simulink library "ammclib_bam_s32k14x"  (Simulink 9.0)
settings: Solver=ode45  StartTime=0.0  StopTime=10.0  RelTol=1e-3
undefined symbols (not defined in the file): f16A1, f16A2, f16B0, f16B1, f16B2, f16C1, f16CC1, f16CC1sc, f16CC1sc_D, f16CC1sc_Q, f16CC1scD, f16CC1scQ, f16CC2, f16CC2sc, f16CC2sc_D, f16CC2sc_Q, f16CC2scD, f16CC2scQ, f16DerivGain, f16EGain, f16FiltCoef, f16HystOff, f16HystOn, f16IGain, f16IntegGain, f16IntegGainFW, f16IntegGainQ, f16Kd, f16Kq, f16Limit, f16LowerLim, f16LowerLimit_D, f16LowerLimit_Q, f16ModIndex, f16OutValOff, f16OutValOn, f16PropGain, f16PropGainFW, f16PropGainQ, f16RampDown, f16RampUp, f16UGain, f16UpperLim, f16UpperLimit, f16UpperLimit_D, f16UpperLimit_Q, f16WIGain, f32A1, f32A2, f32B0, f32B1, f32B2, f32C1, f32CC1, f32CC1sc, f32CC1sc_D, f32CC1sc_Q, f32CC1scD, f32CC1scQ, f32CC2 ... (+122)
(part 10 of 11)

== system ammclib_bam_s32k14x/MLIB/bam_flt/MLIB_Mul_FLT ==
  note: ---------------------------------------------------------------------------------------------------------------------------------------------------------------------------------------------------
  fltIn1 : Inport
  fltIn2 : Inport  Port=2
  MLIB_Mul_SF : S-Function  FunctionName=MLIB_Mul_SF_FLT  SFunctionDeploymentMode=off  EnableBusSupport=off
  copyright : Subsystem
      mask Display:
      | text(10,90,'FILE:');text(10,75,'DESRIPTION:')
      | text(10,60,'COPYRIGHT:')
      | text(10,45,'VERSION:')
      | text(10,30,'DATE:')
  copyright2 : Subsystem
      mask Display:
      | text(10,90,'MLIB_Mul_BAM_FLT.mdl');text(10,75,'Sum of two input values.');text(10,60,'NXP')
      | text(10,45,'0.1');text(10,30,'26-Jul-2011');
  logo : Subsystem
      mask Display: image(imread('logo.jpg'))
  fltOut : Outport
  wires:
  MLIB_Mul_SF/1 -> fltOut/1
  fltIn2/1 -> MLIB_Mul_SF/2
  fltIn1/1 -> MLIB_Mul_SF/1

== system ammclib_bam_s32k14x/MLIB/bam_flt/MLIB_Neg_FLT ==
  note: ---------------------------------------------------------------------------------------------------------------------------------------------------------------------------------------------------
  fltIn : Inport
  MLIB_Neg_SF : S-Function  FunctionName=MLIB_Neg_SF_FLT  SFunctionDeploymentMode=off  EnableBusSupport=off
  copyright : Subsystem
      mask Display:
      | text(10,90,'FILE:');text(10,75,'DESRIPTION:')
      | text(10,60,'COPYRIGHT:')
      | text(10,45,'VERSION:')
      | text(10,30,'DATE:')
  copyright2 : Subsystem
      mask Display:
      | text(10,90,'MLIB_Neg_BAM_FLT.mdl');text(10,75,'Sum of two input values.');text(10,60,'NXP')
      | text(10,45,'0.1');text(10,30,'20-Jan-2012');
  logo : Subsystem
      mask Display: image(imread('logo.jpg'))
  fltOut : Outport
  wires:
  MLIB_Neg_SF/1 -> fltOut/1
  fltIn/1 -> MLIB_Neg_SF/1

== system ammclib_bam_s32k14x/MLIB/bam_flt/MLIB_Sub_FLT ==
  note: ---------------------------------------------------------------------------------------------------------------------------------------------------------------------------------------------------
  fltIn1 : Inport
  fltIn2 : Inport  Port=2
  MLIB_Sub_SF : S-Function  FunctionName=MLIB_Sub_SF_FLT  SFunctionDeploymentMode=off  EnableBusSupport=off
  copyright : Subsystem
      mask Display:
      | text(10,90,'FILE:');text(10,75,'DESRIPTION:')
      | text(10,60,'COPYRIGHT:')
      | text(10,45,'VERSION:')
      | text(10,30,'DATE:')
  copyright2 : Subsystem
      mask Display:
      | text(10,90,'MLIB_Sub_BAM_FLT.mdl');text(10,75,'Sum of two input values.');text(10,60,'NXP')
      | text(10,45,'0.1');text(10,30,'18-Jul-2011');
  logo : Subsystem
      mask Display: image(imread('logo.jpg'))
  fltOut : Outport
  wires:
  MLIB_Sub_SF/1 -> fltOut/1
  fltIn2/1 -> MLIB_Sub_SF/2
  fltIn1/1 -> MLIB_Sub_SF/1

== system ammclib_bam_s32k14x/MLIB/bam_flt/MLIB_VMac_FLT ==
  note: ---------------------------------------------------------------------------------------------------------------------------------------------------------------------------------------------------
  fltIn1 : Inport
  fltIn2 : Inport  Port=2
  fltIn3 : Inport  Port=3
  fltIn4 : Inport  Port=4
  MLIB_VMac_SF : S-Function  FunctionName=MLIB_VMac_SF_FLT  SFunctionDeploymentMode=off  EnableBusSupport=off
  copyright : Subsystem
      mask Display:
      | text(10,90,'FILE:');text(10,75,'DESRIPTION:')
      | text(10,60,'COPYRIGHT:')
      | text(10,45,'VERSION:')
      | text(10,30,'DATE:')
  copyright2 : Subsystem
      mask Display:
      | text(10,90,'MLIB_VMac_BAM_FLT.mdl');text(10,75,'Vector multiply accumulate.');text(10,60,'Freescale')
      | text(10,45,'0.1');text(10,30,'25-Aug-2011');
  logo : Subsystem
      mask Display: image(imread('logo.jpg'))
  fltOut : Outport
  wires:
  MLIB_VMac_SF/1 -> fltOut/1
  fltIn4/1 -> MLIB_VMac_SF/4
  fltIn3/1 -> MLIB_VMac_SF/3
  fltIn2/1 -> MLIB_VMac_SF/2
  fltIn1/1 -> MLIB_VMac_SF/1

== system ammclib_bam_s32k14x/AMCLIB/bam_f16/AMCLIB_BemfObsrvDQ_F16/copyright ==

== system ammclib_bam_s32k14x/AMCLIB/bam_f16/AMCLIB_BemfObsrvDQ_F16/copyright2 ==

== system ammclib_bam_s32k14x/AMCLIB/bam_f16/AMCLIB_BemfObsrvDQ_F16/logo ==

== system ammclib_bam_s32k14x/AMCLIB/bam_f16/AMCLIB_CurrentLoop_F16/copyright ==

== system ammclib_bam_s32k14x/AMCLIB/bam_f16/AMCLIB_CurrentLoop_F16/copyright2 ==

== system ammclib_bam_s32k14x/AMCLIB/bam_f16/AMCLIB_CurrentLoop_F16/logo ==

== system ammclib_bam_s32k14x/AMCLIB/bam_f16/AMCLIB_FWSpeedLoop_F16/copyright ==

== system ammclib_bam_s32k14x/AMCLIB/bam_f16/AMCLIB_FWSpeedLoop_F16/copyright2 ==

== system ammclib_bam_s32k14x/AMCLIB/bam_f16/AMCLIB_FWSpeedLoop_F16/logo ==

== system ammclib_bam_s32k14x/AMCLIB/bam_f16/AMCLIB_FW_F16/copyright ==

== system ammclib_bam_s32k14x/AMCLIB/bam_f16/AMCLIB_FW_F16/copyright2 ==

== system ammclib_bam_s32k14x/AMCLIB/bam_f16/AMCLIB_FW_F16/logo ==

== system ammclib_bam_s32k14x/AMCLIB/bam_f16/AMCLIB_SpeedLoop_F16/copyright ==

== system ammclib_bam_s32k14x/AMCLIB/bam_f16/AMCLIB_SpeedLoop_F16/copyright2 ==

== system ammclib_bam_s32k14x/AMCLIB/bam_f16/AMCLIB_SpeedLoop_F16/logo ==

== system ammclib_bam_s32k14x/AMCLIB/bam_f16/AMCLIB_TrackObsrv_F16/copyright ==

== system ammclib_bam_s32k14x/AMCLIB/bam_f16/AMCLIB_TrackObsrv_F16/copyright2 ==

== system ammclib_bam_s32k14x/AMCLIB/bam_f16/AMCLIB_TrackObsrv_F16/logo ==

== system ammclib_bam_s32k14x/AMCLIB/bam_f32/AMCLIB_BemfObsrvDQ_F32/copyright ==

== system ammclib_bam_s32k14x/AMCLIB/bam_f32/AMCLIB_BemfObsrvDQ_F32/copyright2 ==

== system ammclib_bam_s32k14x/AMCLIB/bam_f32/AMCLIB_BemfObsrvDQ_F32/logo ==

== system ammclib_bam_s32k14x/AMCLIB/bam_f32/AMCLIB_CurrentLoop_F32/copyright ==

== system ammclib_bam_s32k14x/AMCLIB/bam_f32/AMCLIB_CurrentLoop_F32/copyright2 ==

== system ammclib_bam_s32k14x/AMCLIB/bam_f32/AMCLIB_CurrentLoop_F32/logo ==

== system ammclib_bam_s32k14x/AMCLIB/bam_f32/AMCLIB_FWSpeedLoop_F32/copyright ==

== system ammclib_bam_s32k14x/AMCLIB/bam_f32/AMCLIB_FWSpeedLoop_F32/copyright2 ==

== system ammclib_bam_s32k14x/AMCLIB/bam_f32/AMCLIB_FWSpeedLoop_F32/logo ==

== system ammclib_bam_s32k14x/AMCLIB/bam_f32/AMCLIB_FW_F32/copyright ==

== system ammclib_bam_s32k14x/AMCLIB/bam_f32/AMCLIB_FW_F32/copyright2 ==

== system ammclib_bam_s32k14x/AMCLIB/bam_f32/AMCLIB_FW_F32/logo ==

== system ammclib_bam_s32k14x/AMCLIB/bam_f32/AMCLIB_SpeedLoop_F32/copyright ==

== system ammclib_bam_s32k14x/AMCLIB/bam_f32/AMCLIB_SpeedLoop_F32/copyright2 ==

== system ammclib_bam_s32k14x/AMCLIB/bam_f32/AMCLIB_SpeedLoop_F32/logo ==

== system ammclib_bam_s32k14x/AMCLIB/bam_f32/AMCLIB_TrackObsrv_F32/copyright ==

== system ammclib_bam_s32k14x/AMCLIB/bam_f32/AMCLIB_TrackObsrv_F32/copyright2 ==

== system ammclib_bam_s32k14x/AMCLIB/bam_f32/AMCLIB_TrackObsrv_F32/logo ==

== system ammclib_bam_s32k14x/AMCLIB/bam_flt/AMCLIB_BemfObsrvDQ_FLT/copyright ==

== system ammclib_bam_s32k14x/AMCLIB/bam_flt/AMCLIB_BemfObsrvDQ_FLT/copyright2 ==

== system ammclib_bam_s32k14x/AMCLIB/bam_flt/AMCLIB_BemfObsrvDQ_FLT/logo ==

== system ammclib_bam_s32k14x/AMCLIB/bam_flt/AMCLIB_CurrentLoop_FLT/copyright ==

== system ammclib_bam_s32k14x/AMCLIB/bam_flt/AMCLIB_CurrentLoop_FLT/copyright2 ==

== system ammclib_bam_s32k14x/AMCLIB/bam_flt/AMCLIB_CurrentLoop_FLT/logo ==

== system ammclib_bam_s32k14x/AMCLIB/bam_flt/AMCLIB_FWSpeedLoop_FLT/copyright ==

== system ammclib_bam_s32k14x/AMCLIB/bam_flt/AMCLIB_FWSpeedLoop_FLT/copyright2 ==

== system ammclib_bam_s32k14x/AMCLIB/bam_flt/AMCLIB_FWSpeedLoop_FLT/logo ==

== system ammclib_bam_s32k14x/AMCLIB/bam_flt/AMCLIB_FW_FLT/copyright ==

== system ammclib_bam_s32k14x/AMCLIB/bam_flt/AMCLIB_FW_FLT/copyright2 ==

== system ammclib_bam_s32k14x/AMCLIB/bam_flt/AMCLIB_FW_FLT/logo ==

== system ammclib_bam_s32k14x/AMCLIB/bam_flt/AMCLIB_SpeedLoop_FLT/copyright ==

== system ammclib_bam_s32k14x/AMCLIB/bam_flt/AMCLIB_SpeedLoop_FLT/copyright2 ==

== system ammclib_bam_s32k14x/AMCLIB/bam_flt/AMCLIB_SpeedLoop_FLT/logo ==

== system ammclib_bam_s32k14x/AMCLIB/bam_flt/AMCLIB_TrackObsrv_FLT/copyright ==

== system ammclib_bam_s32k14x/AMCLIB/bam_flt/AMCLIB_TrackObsrv_FLT/copyright2 ==

== system ammclib_bam_s32k14x/AMCLIB/bam_flt/AMCLIB_TrackObsrv_FLT/logo ==

== system ammclib_bam_s32k14x/GDFLIB/bam_f16/GDFLIB_FilterFIR_F16/copyright ==

== system ammclib_bam_s32k14x/GDFLIB/bam_f16/GDFLIB_FilterFIR_F16/copyright2 ==

== system ammclib_bam_s32k14x/GDFLIB/bam_f16/GDFLIB_FilterFIR_F16/logo ==

== system ammclib_bam_s32k14x/GDFLIB/bam_f16/GDFLIB_FilterIIR1_F16/copyright ==

== system ammclib_bam_s32k14x/GDFLIB/bam_f16/GDFLIB_FilterIIR1_F16/copyright2 ==

== system ammclib_bam_s32k14x/GDFLIB/bam_f16/GDFLIB_FilterIIR1_F16/logo ==

== system ammclib_bam_s32k14x/GDFLIB/bam_f16/GDFLIB_FilterIIR2_F16/copyright ==

== system ammclib_bam_s32k14x/GDFLIB/bam_f16/GDFLIB_FilterIIR2_F16/copyright2 ==

== system ammclib_bam_s32k14x/GDFLIB/bam_f16/GDFLIB_FilterIIR2_F16/logo ==

== system ammclib_bam_s32k14x/GDFLIB/bam_f16/GDFLIB_FilterMA_F16/copyright ==

== system ammclib_bam_s32k14x/GDFLIB/bam_f16/GDFLIB_FilterMA_F16/copyright2 ==

== system ammclib_bam_s32k14x/GDFLIB/bam_f16/GDFLIB_FilterMA_F16/logo ==

== system ammclib_bam_s32k14x/GDFLIB/bam_f32/GDFLIB_FilterFIR_F32/copyright ==

== system ammclib_bam_s32k14x/GDFLIB/bam_f32/GDFLIB_FilterFIR_F32/copyright2 ==

== system ammclib_bam_s32k14x/GDFLIB/bam_f32/GDFLIB_FilterFIR_F32/logo ==

== system ammclib_bam_s32k14x/GDFLIB/bam_f32/GDFLIB_FilterIIR1_F32/copyright ==

== system ammclib_bam_s32k14x/GDFLIB/bam_f32/GDFLIB_FilterIIR1_F32/copyright2 ==

== system ammclib_bam_s32k14x/GDFLIB/bam_f32/GDFLIB_FilterIIR1_F32/logo ==

== system ammclib_bam_s32k14x/GDFLIB/bam_f32/GDFLIB_FilterIIR2_F32/copyright ==

== system ammclib_bam_s32k14x/GDFLIB/bam_f32/GDFLIB_FilterIIR2_F32/copyright2 ==

== system ammclib_bam_s32k14x/GDFLIB/bam_f32/GDFLIB_FilterIIR2_F32/logo ==

== system ammclib_bam_s32k14x/GDFLIB/bam_f32/GDFLIB_FilterMA_F32/copyright ==

== system ammclib_bam_s32k14x/GDFLIB/bam_f32/GDFLIB_FilterMA_F32/copyright2 ==

== system ammclib_bam_s32k14x/GDFLIB/bam_f32/GDFLIB_FilterMA_F32/logo ==

== system ammclib_bam_s32k14x/GDFLIB/bam_flt/GDFLIB_FilterFIR_FLT/copyright ==

== system ammclib_bam_s32k14x/GDFLIB/bam_flt/GDFLIB_FilterFIR_FLT/copyright2 ==

== system ammclib_bam_s32k14x/GDFLIB/bam_flt/GDFLIB_FilterFIR_FLT/logo ==

== system ammclib_bam_s32k14x/GDFLIB/bam_flt/GDFLIB_FilterIIR1_FLT/copyright ==

== system ammclib_bam_s32k14x/GDFLIB/bam_flt/GDFLIB_FilterIIR1_FLT/copyright2 ==

== system ammclib_bam_s32k14x/GDFLIB/bam_flt/GDFLIB_FilterIIR1_FLT/logo ==

== system ammclib_bam_s32k14x/GDFLIB/bam_flt/GDFLIB_FilterIIR2_FLT/copyright ==

== system ammclib_bam_s32k14x/GDFLIB/bam_flt/GDFLIB_FilterIIR2_FLT/copyright2 ==

== system ammclib_bam_s32k14x/GDFLIB/bam_flt/GDFLIB_FilterIIR2_FLT/logo ==

== system ammclib_bam_s32k14x/GDFLIB/bam_flt/GDFLIB_FilterMA_FLT/copyright ==

== system ammclib_bam_s32k14x/GDFLIB/bam_flt/GDFLIB_FilterMA_FLT/copyright2 ==

== system ammclib_bam_s32k14x/GDFLIB/bam_flt/GDFLIB_FilterMA_FLT/logo ==

== system ammclib_bam_s32k14x/GFLIB/bam_f16/GFLIB_Acos_F16/copyright ==

== system ammclib_bam_s32k14x/GFLIB/bam_f16/GFLIB_Acos_F16/copyright2 ==

== system ammclib_bam_s32k14x/GFLIB/bam_f16/GFLIB_Acos_F16/logo ==

== system ammclib_bam_s32k14x/GFLIB/bam_f16/GFLIB_Asin_F16/copyright ==

== system ammclib_bam_s32k14x/GFLIB/bam_f16/GFLIB_Asin_F16/copyright2 ==

== system ammclib_bam_s32k14x/GFLIB/bam_f16/GFLIB_Asin_F16/logo ==

== system ammclib_bam_s32k14x/GFLIB/bam_f16/GFLIB_AtanYXShifted_F16/copyright ==

== system ammclib_bam_s32k14x/GFLIB/bam_f16/GFLIB_AtanYXShifted_F16/copyright2 ==

== system ammclib_bam_s32k14x/GFLIB/bam_f16/GFLIB_AtanYXShifted_F16/logo ==

== system ammclib_bam_s32k14x/GFLIB/bam_f16/GFLIB_AtanYX_F16/copyright ==

== system ammclib_bam_s32k14x/GFLIB/bam_f16/GFLIB_AtanYX_F16/copyright2 ==

== system ammclib_bam_s32k14x/GFLIB/bam_f16/GFLIB_AtanYX_F16/logo ==

== system ammclib_bam_s32k14x/GFLIB/bam_f16/GFLIB_Atan_F16/copyright ==

== system ammclib_bam_s32k14x/GFLIB/bam_f16/GFLIB_Atan_F16/copyright2 ==

== system ammclib_bam_s32k14x/GFLIB/bam_f16/GFLIB_Atan_F16/logo ==

== system ammclib_bam_s32k14x/GFLIB/bam_f16/GFLIB_ControllerPIDpAW_F16/copyright ==

== system ammclib_bam_s32k14x/GFLIB/bam_f16/GFLIB_ControllerPIDpAW_F16/copyright2 ==

== system ammclib_bam_s32k14x/GFLIB/bam_f16/GFLIB_ControllerPIDpAW_F16/logo ==

== system ammclib_bam_s32k14x/GFLIB/bam_f16/GFLIB_ControllerPIpAW_F16/copyright ==

== system ammclib_bam_s32k14x/GFLIB/bam_f16/GFLIB_ControllerPIpAW_F16/copyright2 ==

== system ammclib_bam_s32k14x/GFLIB/bam_f16/GFLIB_ControllerPIpAW_F16/logo ==

== system ammclib_bam_s32k14x/GFLIB/bam_f16/GFLIB_ControllerPIp_F16/copyright ==

== system ammclib_bam_s32k14x/GFLIB/bam_f16/GFLIB_ControllerPIp_F16/copyright2 ==

== system ammclib_bam_s32k14x/GFLIB/bam_f16/GFLIB_ControllerPIp_F16/logo ==

== system ammclib_bam_s32k14x/GFLIB/bam_f16/GFLIB_ControllerPIrAW_F16/copyright ==

== system ammclib_bam_s32k14x/GFLIB/bam_f16/GFLIB_ControllerPIrAW_F16/copyright2 ==

== system ammclib_bam_s32k14x/GFLIB/bam_f16/GFLIB_ControllerPIrAW_F16/logo ==

== system ammclib_bam_s32k14x/GFLIB/bam_f16/GFLIB_ControllerPIr_F16/copyright ==

== system ammclib_bam_s32k14x/GFLIB/bam_f16/GFLIB_ControllerPIr_F16/copyright2 ==

== system ammclib_bam_s32k14x/GFLIB/bam_f16/GFLIB_ControllerPIr_F16/logo ==

== system ammclib_bam_s32k14x/GFLIB/bam_f16/GFLIB_Cos_F16/copyright ==

== system ammclib_bam_s32k14x/GFLIB/bam_f16/GFLIB_Cos_F16/copyright2 ==

== system ammclib_bam_s32k14x/GFLIB/bam_f16/GFLIB_Cos_F16/logo ==

== system ammclib_bam_s32k14x/GFLIB/bam_f16/GFLIB_Hyst_F16/copyright ==

== system ammclib_bam_s32k14x/GFLIB/bam_f16/GFLIB_Hyst_F16/copyright2 ==

== system ammclib_bam_s32k14x/GFLIB/bam_f16/GFLIB_Hyst_F16/logo ==

== system ammclib_bam_s32k14x/GFLIB/bam_f16/GFLIB_IntegratorTR_F16/copyright ==

== system ammclib_bam_s32k14x/GFLIB/bam_f16/GFLIB_IntegratorTR_F16/copyright2 ==

== system ammclib_bam_s32k14x/GFLIB/bam_f16/GFLIB_IntegratorTR_F16/logo ==

== system ammclib_bam_s32k14x/GFLIB/bam_f16/GFLIB_Limit_F16/copyright ==

== system ammclib_bam_s32k14x/GFLIB/bam_f16/GFLIB_Limit_F16/copyright2 ==

== system ammclib_bam_s32k14x/GFLIB/bam_f16/GFLIB_Limit_F16/logo ==

== system ammclib_bam_s32k14x/GFLIB/bam_f16/GFLIB_LowerLimit_F16/copyright ==

== system ammclib_bam_s32k14x/GFLIB/bam_f16/GFLIB_LowerLimit_F16/copyright2 ==

== system ammclib_bam_s32k14x/GFLIB/bam_f16/GFLIB_LowerLimit_F16/logo ==

== system ammclib_bam_s32k14x/GFLIB/bam_f16/GFLIB_Lut1D_F16/copyright ==

== system ammclib_bam_s32k14x/GFLIB/bam_f16/GFLIB_Lut1D_F16/copyright2 ==

== system ammclib_bam_s32k14x/GFLIB/bam_f16/GFLIB_Lut1D_F16/logo ==

== system ammclib_bam_s32k14x/GFLIB/bam_f16/GFLIB_Lut2D_F16/copyright ==

== system ammclib_bam_s32k14x/GFLIB/bam_f16/GFLIB_Lut2D_F16/copyright2 ==

== system ammclib_bam_s32k14x/GFLIB/bam_f16/GFLIB_Lut2D_F16/logo ==

== system ammclib_bam_s32k14x/GFLIB/bam_f16/GFLIB_Ramp_F16/copyright ==

== system ammclib_bam_s32k14x/GFLIB/bam_f16/GFLIB_Ramp_F16/copyright2 ==

== system ammclib_bam_s32k14x/GFLIB/bam_f16/GFLIB_Ramp_F16/logo ==

== system ammclib_bam_s32k14x/GFLIB/bam_f16/GFLIB_Sign_F16/copyright ==

== system ammclib_bam_s32k14x/GFLIB/bam_f16/GFLIB_Sign_F16/copyright2 ==

== system ammclib_bam_s32k14x/GFLIB/bam_f16/GFLIB_Sign_F16/logo ==

== system ammclib_bam_s32k14x/GFLIB/bam_f16/GFLIB_SinCos_F16/copyright ==

== system ammclib_bam_s32k14x/GFLIB/bam_f16/GFLIB_SinCos_F16/copyright2 ==

== system ammclib_bam_s32k14x/GFLIB/bam_f16/GFLIB_SinCos_F16/logo ==

== system ammclib_bam_s32k14x/GFLIB/bam_f16/GFLIB_Sin_F16/copyright ==

== system ammclib_bam_s32k14x/GFLIB/bam_f16/GFLIB_Sin_F16/copyright2 ==

== system ammclib_bam_s32k14x/GFLIB/bam_f16/GFLIB_Sin_F16/logo ==

== system ammclib_bam_s32k14x/GFLIB/bam_f16/GFLIB_Sqrt_F16/copyright ==

== system ammclib_bam_s32k14x/GFLIB/bam_f16/GFLIB_Sqrt_F16/copyright2 ==

== system ammclib_bam_s32k14x/GFLIB/bam_f16/GFLIB_Sqrt_F16/logo ==

== system ammclib_bam_s32k14x/GFLIB/bam_f16/GFLIB_Tan_F16/copyright ==

== system ammclib_bam_s32k14x/GFLIB/bam_f16/GFLIB_Tan_F16/copyright2 ==

== system ammclib_bam_s32k14x/GFLIB/bam_f16/GFLIB_Tan_F16/logo ==

== system ammclib_bam_s32k14x/GFLIB/bam_f16/GFLIB_UpperLimit_F16/copyright ==

== system ammclib_bam_s32k14x/GFLIB/bam_f16/GFLIB_UpperLimit_F16/copyright2 ==

== system ammclib_bam_s32k14x/GFLIB/bam_f16/GFLIB_UpperLimit_F16/logo ==

== system ammclib_bam_s32k14x/GFLIB/bam_f16/GFLIB_VMin_F16/copyright ==

== system ammclib_bam_s32k14x/GFLIB/bam_f16/GFLIB_VMin_F16/copyright2 ==

== system ammclib_bam_s32k14x/GFLIB/bam_f16/GFLIB_VMin_F16/logo ==

== system ammclib_bam_s32k14x/GFLIB/bam_f16/GFLIB_VectorLimit_F16/copyright ==

== system ammclib_bam_s32k14x/GFLIB/bam_f16/GFLIB_VectorLimit_F16/copyright2 ==

== system ammclib_bam_s32k14x/GFLIB/bam_f16/GFLIB_VectorLimit_F16/logo ==

== system ammclib_bam_s32k14x/GFLIB/bam_f32/GFLIB_Acos_F32/copyright ==

== system ammclib_bam_s32k14x/GFLIB/bam_f32/GFLIB_Acos_F32/copyright2 ==

== system ammclib_bam_s32k14x/GFLIB/bam_f32/GFLIB_Acos_F32/logo ==

== system ammclib_bam_s32k14x/GFLIB/bam_f32/GFLIB_Asin_F32/copyright ==

== system ammclib_bam_s32k14x/GFLIB/bam_f32/GFLIB_Asin_F32/copyright2 ==

== system ammclib_bam_s32k14x/GFLIB/bam_f32/GFLIB_Asin_F32/logo ==

== system ammclib_bam_s32k14x/GFLIB/bam_f32/GFLIB_AtanYXShifted_F32/copyright ==

== system ammclib_bam_s32k14x/GFLIB/bam_f32/GFLIB_AtanYXShifted_F32/copyright2 ==

== system ammclib_bam_s32k14x/GFLIB/bam_f32/GFLIB_AtanYXShifted_F32/logo ==

== system ammclib_bam_s32k14x/GFLIB/bam_f32/GFLIB_AtanYX_F32/copyright ==

== system ammclib_bam_s32k14x/GFLIB/bam_f32/GFLIB_AtanYX_F32/copyright2 ==

== system ammclib_bam_s32k14x/GFLIB/bam_f32/GFLIB_AtanYX_F32/logo ==

== system ammclib_bam_s32k14x/GFLIB/bam_f32/GFLIB_Atan_F32/copyright ==

== system ammclib_bam_s32k14x/GFLIB/bam_f32/GFLIB_Atan_F32/copyright2 ==

== system ammclib_bam_s32k14x/GFLIB/bam_f32/GFLIB_Atan_F32/logo ==

== system ammclib_bam_s32k14x/GFLIB/bam_f32/GFLIB_ControllerPIDpAW_F32/copyright ==

== system ammclib_bam_s32k14x/GFLIB/bam_f32/GFLIB_ControllerPIDpAW_F32/copyright2 ==

== system ammclib_bam_s32k14x/GFLIB/bam_f32/GFLIB_ControllerPIDpAW_F32/logo ==

== system ammclib_bam_s32k14x/GFLIB/bam_f32/GFLIB_ControllerPIpAW_F32/copyright ==

== system ammclib_bam_s32k14x/GFLIB/bam_f32/GFLIB_ControllerPIpAW_F32/copyright2 ==

== system ammclib_bam_s32k14x/GFLIB/bam_f32/GFLIB_ControllerPIpAW_F32/logo ==

== system ammclib_bam_s32k14x/GFLIB/bam_f32/GFLIB_ControllerPIp_F32/copyright ==

== system ammclib_bam_s32k14x/GFLIB/bam_f32/GFLIB_ControllerPIp_F32/copyright2 ==

== system ammclib_bam_s32k14x/GFLIB/bam_f32/GFLIB_ControllerPIp_F32/logo ==

== system ammclib_bam_s32k14x/GFLIB/bam_f32/GFLIB_ControllerPIrAW_F32/copyright ==

== system ammclib_bam_s32k14x/GFLIB/bam_f32/GFLIB_ControllerPIrAW_F32/copyright2 ==

== system ammclib_bam_s32k14x/GFLIB/bam_f32/GFLIB_ControllerPIrAW_F32/logo ==

== system ammclib_bam_s32k14x/GFLIB/bam_f32/GFLIB_ControllerPIr_F32/copyright ==

== system ammclib_bam_s32k14x/GFLIB/bam_f32/GFLIB_ControllerPIr_F32/copyright2 ==

== system ammclib_bam_s32k14x/GFLIB/bam_f32/GFLIB_ControllerPIr_F32/logo ==

== system ammclib_bam_s32k14x/GFLIB/bam_f32/GFLIB_Cos_F32/copyright ==

== system ammclib_bam_s32k14x/GFLIB/bam_f32/GFLIB_Cos_F32/copyright2 ==

== system ammclib_bam_s32k14x/GFLIB/bam_f32/GFLIB_Cos_F32/logo ==

== system ammclib_bam_s32k14x/GFLIB/bam_f32/GFLIB_Hyst_F32/copyright ==

== system ammclib_bam_s32k14x/GFLIB/bam_f32/GFLIB_Hyst_F32/copyright2 ==

== system ammclib_bam_s32k14x/GFLIB/bam_f32/GFLIB_Hyst_F32/logo ==

== system ammclib_bam_s32k14x/GFLIB/bam_f32/GFLIB_IntegratorTR_F32/copyright ==

== system ammclib_bam_s32k14x/GFLIB/bam_f32/GFLIB_IntegratorTR_F32/copyright2 ==

== system ammclib_bam_s32k14x/GFLIB/bam_f32/GFLIB_IntegratorTR_F32/logo ==

== system ammclib_bam_s32k14x/GFLIB/bam_f32/GFLIB_Limit_F32/copyright ==

== system ammclib_bam_s32k14x/GFLIB/bam_f32/GFLIB_Limit_F32/copyright2 ==

== system ammclib_bam_s32k14x/GFLIB/bam_f32/GFLIB_Limit_F32/logo ==

== system ammclib_bam_s32k14x/GFLIB/bam_f32/GFLIB_LowerLimit_F32/copyright ==

== system ammclib_bam_s32k14x/GFLIB/bam_f32/GFLIB_LowerLimit_F32/copyright2 ==

== system ammclib_bam_s32k14x/GFLIB/bam_f32/GFLIB_LowerLimit_F32/logo ==

== system ammclib_bam_s32k14x/GFLIB/bam_f32/GFLIB_Lut1D_F32/copyright ==

== system ammclib_bam_s32k14x/GFLIB/bam_f32/GFLIB_Lut1D_F32/copyright2 ==

== system ammclib_bam_s32k14x/GFLIB/bam_f32/GFLIB_Lut1D_F32/logo ==

== system ammclib_bam_s32k14x/GFLIB/bam_f32/GFLIB_Lut2D_F32/copyright ==

== system ammclib_bam_s32k14x/GFLIB/bam_f32/GFLIB_Lut2D_F32/copyright2 ==

== system ammclib_bam_s32k14x/GFLIB/bam_f32/GFLIB_Lut2D_F32/logo ==

== system ammclib_bam_s32k14x/GFLIB/bam_f32/GFLIB_Ramp_F32/copyright ==

== system ammclib_bam_s32k14x/GFLIB/bam_f32/GFLIB_Ramp_F32/copyright2 ==

== system ammclib_bam_s32k14x/GFLIB/bam_f32/GFLIB_Ramp_F32/logo ==

== system ammclib_bam_s32k14x/GFLIB/bam_f32/GFLIB_Sign_F32/copyright ==

== system ammclib_bam_s32k14x/GFLIB/bam_f32/GFLIB_Sign_F32/copyright2 ==

== system ammclib_bam_s32k14x/GFLIB/bam_f32/GFLIB_Sign_F32/logo ==

== system ammclib_bam_s32k14x/GFLIB/bam_f32/GFLIB_SinCos_F32/copyright ==

== system ammclib_bam_s32k14x/GFLIB/bam_f32/GFLIB_SinCos_F32/copyright2 ==

== system ammclib_bam_s32k14x/GFLIB/bam_f32/GFLIB_SinCos_F32/logo ==

== system ammclib_bam_s32k14x/GFLIB/bam_f32/GFLIB_Sin_F32/copyright ==

== system ammclib_bam_s32k14x/GFLIB/bam_f32/GFLIB_Sin_F32/copyright2 ==

== system ammclib_bam_s32k14x/GFLIB/bam_f32/GFLIB_Sin_F32/logo ==

== system ammclib_bam_s32k14x/GFLIB/bam_f32/GFLIB_Sqrt_F32/copyright ==

== system ammclib_bam_s32k14x/GFLIB/bam_f32/GFLIB_Sqrt_F32/copyright2 ==

== system ammclib_bam_s32k14x/GFLIB/bam_f32/GFLIB_Sqrt_F32/logo ==

== system ammclib_bam_s32k14x/GFLIB/bam_f32/GFLIB_Tan_F32/copyright ==

== system ammclib_bam_s32k14x/GFLIB/bam_f32/GFLIB_Tan_F32/copyright2 ==

== system ammclib_bam_s32k14x/GFLIB/bam_f32/GFLIB_Tan_F32/logo ==

== system ammclib_bam_s32k14x/GFLIB/bam_f32/GFLIB_UpperLimit_F32/copyright ==

== system ammclib_bam_s32k14x/GFLIB/bam_f32/GFLIB_UpperLimit_F32/copyright2 ==

== system ammclib_bam_s32k14x/GFLIB/bam_f32/GFLIB_UpperLimit_F32/logo ==

== system ammclib_bam_s32k14x/GFLIB/bam_f32/GFLIB_VMin_F32/copyright ==

== system ammclib_bam_s32k14x/GFLIB/bam_f32/GFLIB_VMin_F32/copyright2 ==

== system ammclib_bam_s32k14x/GFLIB/bam_f32/GFLIB_VMin_F32/logo ==

== system ammclib_bam_s32k14x/GFLIB/bam_f32/GFLIB_VectorLimit_F32/copyright ==

== system ammclib_bam_s32k14x/GFLIB/bam_f32/GFLIB_VectorLimit_F32/copyright2 ==

== system ammclib_bam_s32k14x/GFLIB/bam_f32/GFLIB_VectorLimit_F32/logo ==

== system ammclib_bam_s32k14x/GFLIB/bam_flt/GFLIB_Acos_FLT/copyright ==

== system ammclib_bam_s32k14x/GFLIB/bam_flt/GFLIB_Acos_FLT/copyright2 ==

== system ammclib_bam_s32k14x/GFLIB/bam_flt/GFLIB_Acos_FLT/logo ==

== system ammclib_bam_s32k14x/GFLIB/bam_flt/GFLIB_Asin_FLT/copyright ==

== system ammclib_bam_s32k14x/GFLIB/bam_flt/GFLIB_Asin_FLT/copyright2 ==

== system ammclib_bam_s32k14x/GFLIB/bam_flt/GFLIB_Asin_FLT/logo ==

== system ammclib_bam_s32k14x/GFLIB/bam_flt/GFLIB_AtanYXShifted_FLT/copyright ==

== system ammclib_bam_s32k14x/GFLIB/bam_flt/GFLIB_AtanYXShifted_FLT/copyright2 ==

== system ammclib_bam_s32k14x/GFLIB/bam_flt/GFLIB_AtanYXShifted_FLT/logo ==

== system ammclib_bam_s32k14x/GFLIB/bam_flt/GFLIB_AtanYX_FLT/copyright ==

== system ammclib_bam_s32k14x/GFLIB/bam_flt/GFLIB_AtanYX_FLT/copyright2 ==

== system ammclib_bam_s32k14x/GFLIB/bam_flt/GFLIB_AtanYX_FLT/logo ==

== system ammclib_bam_s32k14x/GFLIB/bam_flt/GFLIB_Atan_FLT/copyright ==

== system ammclib_bam_s32k14x/GFLIB/bam_flt/GFLIB_Atan_FLT/copyright2 ==

== system ammclib_bam_s32k14x/GFLIB/bam_flt/GFLIB_Atan_FLT/logo ==

== system ammclib_bam_s32k14x/GFLIB/bam_flt/GFLIB_ControllerPIDpAW_FLT/copyright ==

== system ammclib_bam_s32k14x/GFLIB/bam_flt/GFLIB_ControllerPIDpAW_FLT/copyright2 ==

== system ammclib_bam_s32k14x/GFLIB/bam_flt/GFLIB_ControllerPIDpAW_FLT/logo ==

== system ammclib_bam_s32k14x/GFLIB/bam_flt/GFLIB_ControllerPIpAW_FLT/copyright ==

== system ammclib_bam_s32k14x/GFLIB/bam_flt/GFLIB_ControllerPIpAW_FLT/copyright2 ==

== system ammclib_bam_s32k14x/GFLIB/bam_flt/GFLIB_ControllerPIpAW_FLT/logo ==

== system ammclib_bam_s32k14x/GFLIB/bam_flt/GFLIB_ControllerPIp_FLT/copyright ==

== system ammclib_bam_s32k14x/GFLIB/bam_flt/GFLIB_ControllerPIp_FLT/copyright2 ==

== system ammclib_bam_s32k14x/GFLIB/bam_flt/GFLIB_ControllerPIp_FLT/logo ==

== system ammclib_bam_s32k14x/GFLIB/bam_flt/GFLIB_ControllerPIrAW_FLT/copyright ==

== system ammclib_bam_s32k14x/GFLIB/bam_flt/GFLIB_ControllerPIrAW_FLT/copyright2 ==

== system ammclib_bam_s32k14x/GFLIB/bam_flt/GFLIB_ControllerPIrAW_FLT/logo ==

== system ammclib_bam_s32k14x/GFLIB/bam_flt/GFLIB_ControllerPIr_FLT/copyright ==

== system ammclib_bam_s32k14x/GFLIB/bam_flt/GFLIB_ControllerPIr_FLT/copyright2 ==

== system ammclib_bam_s32k14x/GFLIB/bam_flt/GFLIB_ControllerPIr_FLT/logo ==

== system ammclib_bam_s32k14x/GFLIB/bam_flt/GFLIB_Cos_FLT/copyright ==

== system ammclib_bam_s32k14x/GFLIB/bam_flt/GFLIB_Cos_FLT/copyright2 ==

== system ammclib_bam_s32k14x/GFLIB/bam_flt/GFLIB_Cos_FLT/logo ==

== system ammclib_bam_s32k14x/GFLIB/bam_flt/GFLIB_Hyst_FLT/copyright ==

== system ammclib_bam_s32k14x/GFLIB/bam_flt/GFLIB_Hyst_FLT/copyright2 ==

== system ammclib_bam_s32k14x/GFLIB/bam_flt/GFLIB_Hyst_FLT/logo ==

== system ammclib_bam_s32k14x/GFLIB/bam_flt/GFLIB_IntegratorTR_FLT/copyright ==

== system ammclib_bam_s32k14x/GFLIB/bam_flt/GFLIB_IntegratorTR_FLT/copyright2 ==

== system ammclib_bam_s32k14x/GFLIB/bam_flt/GFLIB_IntegratorTR_FLT/logo ==

== system ammclib_bam_s32k14x/GFLIB/bam_flt/GFLIB_Limit_FLT/copyright ==

== system ammclib_bam_s32k14x/GFLIB/bam_flt/GFLIB_Limit_FLT/copyright2 ==

== system ammclib_bam_s32k14x/GFLIB/bam_flt/GFLIB_Limit_FLT/logo ==

== system ammclib_bam_s32k14x/GFLIB/bam_flt/GFLIB_Log10_FLT/copyright ==

== system ammclib_bam_s32k14x/GFLIB/bam_flt/GFLIB_Log10_FLT/copyright2 ==

== system ammclib_bam_s32k14x/GFLIB/bam_flt/GFLIB_Log10_FLT/logo ==

== system ammclib_bam_s32k14x/GFLIB/bam_flt/GFLIB_LowerLimit_FLT/copyright ==

== system ammclib_bam_s32k14x/GFLIB/bam_flt/GFLIB_LowerLimit_FLT/copyright2 ==

== system ammclib_bam_s32k14x/GFLIB/bam_flt/GFLIB_LowerLimit_FLT/logo ==

== system ammclib_bam_s32k14x/GFLIB/bam_flt/GFLIB_Lut1D_FLT/copyright ==

== system ammclib_bam_s32k14x/GFLIB/bam_flt/GFLIB_Lut1D_FLT/copyright2 ==

== system ammclib_bam_s32k14x/GFLIB/bam_flt/GFLIB_Lut1D_FLT/logo ==

== system ammclib_bam_s32k14x/GFLIB/bam_flt/GFLIB_Lut2D_FLT/copyright ==

== system ammclib_bam_s32k14x/GFLIB/bam_flt/GFLIB_Lut2D_FLT/copyright2 ==

== system ammclib_bam_s32k14x/GFLIB/bam_flt/GFLIB_Lut2D_FLT/logo ==

== system ammclib_bam_s32k14x/GFLIB/bam_flt/GFLIB_Ramp_FLT/copyright ==

== system ammclib_bam_s32k14x/GFLIB/bam_flt/GFLIB_Ramp_FLT/copyright2 ==

== system ammclib_bam_s32k14x/GFLIB/bam_flt/GFLIB_Ramp_FLT/logo ==

== system ammclib_bam_s32k14x/GFLIB/bam_flt/GFLIB_Sign_FLT/copyright ==

== system ammclib_bam_s32k14x/GFLIB/bam_flt/GFLIB_Sign_FLT/copyright2 ==

== system ammclib_bam_s32k14x/GFLIB/bam_flt/GFLIB_Sign_FLT/logo ==

== system ammclib_bam_s32k14x/GFLIB/bam_flt/GFLIB_SinCos_FLT/copyright ==

== system ammclib_bam_s32k14x/GFLIB/bam_flt/GFLIB_SinCos_FLT/copyright2 ==

== system ammclib_bam_s32k14x/GFLIB/bam_flt/GFLIB_SinCos_FLT/logo ==

== system ammclib_bam_s32k14x/GFLIB/bam_flt/GFLIB_Sin_FLT/copyright ==

== system ammclib_bam_s32k14x/GFLIB/bam_flt/GFLIB_Sin_FLT/copyright2 ==

== system ammclib_bam_s32k14x/GFLIB/bam_flt/GFLIB_Sin_FLT/logo ==

== system ammclib_bam_s32k14x/GFLIB/bam_flt/GFLIB_Sqrt_FLT/copyright ==

== system ammclib_bam_s32k14x/GFLIB/bam_flt/GFLIB_Sqrt_FLT/copyright2 ==

== system ammclib_bam_s32k14x/GFLIB/bam_flt/GFLIB_Sqrt_FLT/logo ==

== system ammclib_bam_s32k14x/GFLIB/bam_flt/GFLIB_Tan_FLT/copyright ==

== system ammclib_bam_s32k14x/GFLIB/bam_flt/GFLIB_Tan_FLT/copyright2 ==

== system ammclib_bam_s32k14x/GFLIB/bam_flt/GFLIB_Tan_FLT/logo ==

== system ammclib_bam_s32k14x/GFLIB/bam_flt/GFLIB_UpperLimit_FLT/copyright ==

== system ammclib_bam_s32k14x/GFLIB/bam_flt/GFLIB_UpperLimit_FLT/copyright2 ==

== system ammclib_bam_s32k14x/GFLIB/bam_flt/GFLIB_UpperLimit_FLT/logo ==

== system ammclib_bam_s32k14x/GFLIB/bam_flt/GFLIB_VLog10_FLT/GFLIB_VLog10_FLT ==
  note: ---------------------------------------------------------------------------------------------------------------------------------------------------------------------------------------------------
  fltIn : Inport
  GFLIB_VLog10_SF : S-Function  FunctionName=GFLIB_VLog10_SF_FLT  Parameters=u32N  SFunctionDeploymentMode=off  EnableBusSupport=off
  copyright : Subsystem
      mask Display: text(10,90,'FILE:');text(10,75,'DESRIPTION:');text(10,60,'COPYRIGHT:');text(10,45,'VERSION:');text(10,30,'DATE:')
  copyright2 : Subsystem
      mask Display: text(10,90,'GFLIB_VLog10_BAM_FLT.mdl');text(10,75,'Vector fast base-10 logarithm');text(10,60,'NXP');text(10,45,'1.0');text(10,30,'20-Feb-2017');
  logo : Subsystem
      mask Display: image(imread('logo.jpg'))
  fltOut : Outport
  wires:
  GFLIB_VLog10_SF/1 -> fltOut/1
  fltIn/1 -> GFLIB_VLog10_SF/1

== system ammclib_bam_s32k14x/GFLIB/bam_flt/GFLIB_VMin_FLT/copyright ==

== system ammclib_bam_s32k14x/GFLIB/bam_flt/GFLIB_VMin_FLT/copyright2 ==

== system ammclib_bam_s32k14x/GFLIB/bam_flt/GFLIB_VMin_FLT/logo ==

== system ammclib_bam_s32k14x/GFLIB/bam_flt/GFLIB_VectorLimit_FLT/copyright ==

== system ammclib_bam_s32k14x/GFLIB/bam_flt/GFLIB_VectorLimit_FLT/copyright2 ==

== system ammclib_bam_s32k14x/GFLIB/bam_flt/GFLIB_VectorLimit_FLT/logo ==

== system ammclib_bam_s32k14x/GMCLIB/bam_f16/GMCLIB_ClarkInv_F16/copyright ==

== system ammclib_bam_s32k14x/GMCLIB/bam_f16/GMCLIB_ClarkInv_F16/copyright2 ==

== system ammclib_bam_s32k14x/GMCLIB/bam_f16/GMCLIB_ClarkInv_F16/logo ==

== system ammclib_bam_s32k14x/GMCLIB/bam_f16/GMCLIB_Clark_F16/copyright ==

== system ammclib_bam_s32k14x/GMCLIB/bam_f16/GMCLIB_Clark_F16/copyright2 ==

== system ammclib_bam_s32k14x/GMCLIB/bam_f16/GMCLIB_Clark_F16/logo ==

== system ammclib_bam_s32k14x/GMCLIB/bam_f16/GMCLIB_DecouplingPMSM_F16/copyright ==

== system ammclib_bam_s32k14x/GMCLIB/bam_f16/GMCLIB_DecouplingPMSM_F16/copyright2 ==

== system ammclib_bam_s32k14x/GMCLIB/bam_f16/GMCLIB_DecouplingPMSM_F16/logo ==

== system ammclib_bam_s32k14x/GMCLIB/bam_f16/GMCLIB_ElimDcBusRip_F16/copyright ==

== system ammclib_bam_s32k14x/GMCLIB/bam_f16/GMCLIB_ElimDcBusRip_F16/copyright2 ==

== system ammclib_bam_s32k14x/GMCLIB/bam_f16/GMCLIB_ElimDcBusRip_F16/logo ==

== system ammclib_bam_s32k14x/GMCLIB/bam_f16/GMCLIB_ParkInv_F16/copyright ==

== system ammclib_bam_s32k14x/GMCLIB/bam_f16/GMCLIB_ParkInv_F16/copyright2 ==

== system ammclib_bam_s32k14x/GMCLIB/bam_f16/GMCLIB_ParkInv_F16/logo ==

== system ammclib_bam_s32k14x/GMCLIB/bam_f16/GMCLIB_Park_F16/copyright ==

== system ammclib_bam_s32k14x/GMCLIB/bam_f16/GMCLIB_Park_F16/copyright2 ==

== system ammclib_bam_s32k14x/GMCLIB/bam_f16/GMCLIB_Park_F16/logo ==

== system ammclib_bam_s32k14x/GMCLIB/bam_f16/GMCLIB_PwmIct_F16/copyright ==

== system ammclib_bam_s32k14x/GMCLIB/bam_f16/GMCLIB_PwmIct_F16/copyright2 ==

== system ammclib_bam_s32k14x/GMCLIB/bam_f16/GMCLIB_PwmIct_F16/logo ==

== system ammclib_bam_s32k14x/GMCLIB/bam_f16/GMCLIB_SvmStd_F16/copyright ==

== system ammclib_bam_s32k14x/GMCLIB/bam_f16/GMCLIB_SvmStd_F16/copyright2 ==

== system ammclib_bam_s32k14x/GMCLIB/bam_f16/GMCLIB_SvmStd_F16/logo ==

== system ammclib_bam_s32k14x/GMCLIB/bam_f16/GMCLIB_SvmU0n_F16/copyright ==

== system ammclib_bam_s32k14x/GMCLIB/bam_f16/GMCLIB_SvmU0n_F16/copyright2 ==

== system ammclib_bam_s32k14x/GMCLIB/bam_f16/GMCLIB_SvmU0n_F16/logo ==

== system ammclib_bam_s32k14x/GMCLIB/bam_f32/GMCLIB_ClarkInv_F32/copyright ==

== system ammclib_bam_s32k14x/GMCLIB/bam_f32/GMCLIB_ClarkInv_F32/copyright2 ==

== system ammclib_bam_s32k14x/GMCLIB/bam_f32/GMCLIB_ClarkInv_F32/logo ==

== system ammclib_bam_s32k14x/GMCLIB/bam_f32/GMCLIB_Clark_F32/copyright ==

== system ammclib_bam_s32k14x/GMCLIB/bam_f32/GMCLIB_Clark_F32/copyright2 ==

== system ammclib_bam_s32k14x/GMCLIB/bam_f32/GMCLIB_Clark_F32/logo ==

== system ammclib_bam_s32k14x/GMCLIB/bam_f32/GMCLIB_DecouplingPMSM_F32/copyright ==

== system ammclib_bam_s32k14x/GMCLIB/bam_f32/GMCLIB_DecouplingPMSM_F32/copyright2 ==

== system ammclib_bam_s32k14x/GMCLIB/bam_f32/GMCLIB_DecouplingPMSM_F32/logo ==

== system ammclib_bam_s32k14x/GMCLIB/bam_f32/GMCLIB_ElimDcBusRip_F32/copyright ==

== system ammclib_bam_s32k14x/GMCLIB/bam_f32/GMCLIB_ElimDcBusRip_F32/copyright2 ==

== system ammclib_bam_s32k14x/GMCLIB/bam_f32/GMCLIB_ElimDcBusRip_F32/logo ==

== system ammclib_bam_s32k14x/GMCLIB/bam_f32/GMCLIB_ParkInv_F32/copyright ==

== system ammclib_bam_s32k14x/GMCLIB/bam_f32/GMCLIB_ParkInv_F32/copyright2 ==

== system ammclib_bam_s32k14x/GMCLIB/bam_f32/GMCLIB_ParkInv_F32/logo ==

== system ammclib_bam_s32k14x/GMCLIB/bam_f32/GMCLIB_Park_F32/copyright ==

== system ammclib_bam_s32k14x/GMCLIB/bam_f32/GMCLIB_Park_F32/copyright2 ==

== system ammclib_bam_s32k14x/GMCLIB/bam_f32/GMCLIB_Park_F32/logo ==

== system ammclib_bam_s32k14x/GMCLIB/bam_f32/GMCLIB_PwmIct_F32/copyright ==

== system ammclib_bam_s32k14x/GMCLIB/bam_f32/GMCLIB_PwmIct_F32/copyright2 ==

== system ammclib_bam_s32k14x/GMCLIB/bam_f32/GMCLIB_PwmIct_F32/logo ==

== system ammclib_bam_s32k14x/GMCLIB/bam_f32/GMCLIB_SvmStd_F32/copyright ==

== system ammclib_bam_s32k14x/GMCLIB/bam_f32/GMCLIB_SvmStd_F32/copyright2 ==

== system ammclib_bam_s32k14x/GMCLIB/bam_f32/GMCLIB_SvmStd_F32/logo ==

== system ammclib_bam_s32k14x/GMCLIB/bam_f32/GMCLIB_SvmU0n_F32/copyright ==

== system ammclib_bam_s32k14x/GMCLIB/bam_f32/GMCLIB_SvmU0n_F32/copyright2 ==

== system ammclib_bam_s32k14x/GMCLIB/bam_f32/GMCLIB_SvmU0n_F32/logo ==

== system ammclib_bam_s32k14x/GMCLIB/bam_flt/GMCLIB_ClarkInv_FLT/copyright ==

== system ammclib_bam_s32k14x/GMCLIB/bam_flt/GMCLIB_ClarkInv_FLT/copyright2 ==

== system ammclib_bam_s32k14x/GMCLIB/bam_flt/GMCLIB_ClarkInv_FLT/logo ==

== system ammclib_bam_s32k14x/GMCLIB/bam_flt/GMCLIB_Clark_FLT/copyright ==

== system ammclib_bam_s32k14x/GMCLIB/bam_flt/GMCLIB_Clark_FLT/copyright2 ==

== system ammclib_bam_s32k14x/GMCLIB/bam_flt/GMCLIB_Clark_FLT/logo ==

== system ammclib_bam_s32k14x/GMCLIB/bam_flt/GMCLIB_DecouplingPMSM_FLT/copyright ==

== system ammclib_bam_s32k14x/GMCLIB/bam_flt/GMCLIB_DecouplingPMSM_FLT/copyright2 ==

== system ammclib_bam_s32k14x/GMCLIB/bam_flt/GMCLIB_DecouplingPMSM_FLT/logo ==

== system ammclib_bam_s32k14x/GMCLIB/bam_flt/GMCLIB_ElimDcBusRip_FLT/copyright ==

== system ammclib_bam_s32k14x/GMCLIB/bam_flt/GMCLIB_ElimDcBusRip_FLT/copyright2 ==

== system ammclib_bam_s32k14x/GMCLIB/bam_flt/GMCLIB_ElimDcBusRip_FLT/logo ==

== system ammclib_bam_s32k14x/GMCLIB/bam_flt/GMCLIB_ParkInv_FLT/copyright ==

== system ammclib_bam_s32k14x/GMCLIB/bam_flt/GMCLIB_ParkInv_FLT/copyright2 ==

== system ammclib_bam_s32k14x/GMCLIB/bam_flt/GMCLIB_ParkInv_FLT/logo ==

== system ammclib_bam_s32k14x/GMCLIB/bam_flt/GMCLIB_Park_FLT/copyright ==

== system ammclib_bam_s32k14x/GMCLIB/bam_flt/GMCLIB_Park_FLT/copyright2 ==

== system ammclib_bam_s32k14x/GMCLIB/bam_flt/GMCLIB_Park_FLT/logo ==

== system ammclib_bam_s32k14x/GMCLIB/bam_flt/GMCLIB_PwmIct_FLT/copyright ==

== system ammclib_bam_s32k14x/GMCLIB/bam_flt/GMCLIB_PwmIct_FLT/copyright2 ==

== system ammclib_bam_s32k14x/GMCLIB/bam_flt/GMCLIB_PwmIct_FLT/logo ==

== system ammclib_bam_s32k14x/GMCLIB/bam_flt/GMCLIB_SvmStd_FLT/copyright ==

== system ammclib_bam_s32k14x/GMCLIB/bam_flt/GMCLIB_SvmStd_FLT/copyright2 ==

== system ammclib_bam_s32k14x/GMCLIB/bam_flt/GMCLIB_SvmStd_FLT/logo ==

== system ammclib_bam_s32k14x/GMCLIB/bam_flt/GMCLIB_SvmU0n_FLT/copyright ==

== system ammclib_bam_s32k14x/GMCLIB/bam_flt/GMCLIB_SvmU0n_FLT/copyright2 ==

== system ammclib_bam_s32k14x/GMCLIB/bam_flt/GMCLIB_SvmU0n_FLT/logo ==

== system ammclib_bam_s32k14x/MLIB/bam_f16/MLIB_AbsSat_F16/copyright ==

== system ammclib_bam_s32k14x/MLIB/bam_f16/MLIB_AbsSat_F16/copyright2 ==

== system ammclib_bam_s32k14x/MLIB/bam_f16/MLIB_AbsSat_F16/logo ==

== system ammclib_bam_s32k14x/MLIB/bam_f16/MLIB_Abs_F16/copyright ==

== system ammclib_bam_s32k14x/MLIB/bam_f16/MLIB_Abs_F16/copyright2 ==

== system ammclib_bam_s32k14x/MLIB/bam_f16/MLIB_Abs_F16/logo ==

== system ammclib_bam_s32k14x/MLIB/bam_f16/MLIB_AddSat_F16/copyright ==

== system ammclib_bam_s32k14x/MLIB/bam_f16/MLIB_AddSat_F16/copyright2 ==

== system ammclib_bam_s32k14x/MLIB/bam_f16/MLIB_AddSat_F16/logo ==

== system ammclib_bam_s32k14x/MLIB/bam_f16/MLIB_Add_F16/copyright ==

== system ammclib_bam_s32k14x/MLIB/bam_f16/MLIB_Add_F16/copyright2 ==

== system ammclib_bam_s32k14x/MLIB/bam_f16/MLIB_Add_F16/logo ==

== system ammclib_bam_s32k14x/MLIB/bam_f16/MLIB_ConvertPU_F16F32/copyright ==

== system ammclib_bam_s32k14x/MLIB/bam_f16/MLIB_ConvertPU_F16F32/copyright2 ==

== system ammclib_bam_s32k14x/MLIB/bam_f16/MLIB_ConvertPU_F16F32/logo ==

== system ammclib_bam_s32k14x/MLIB/bam_f16/MLIB_ConvertPU_F16FLT/copyright ==

== system ammclib_bam_s32k14x/MLIB/bam_f16/MLIB_ConvertPU_F16FLT/copyright2 ==

== system ammclib_bam_s32k14x/MLIB/bam_f16/MLIB_ConvertPU_F16FLT/logo ==

== system ammclib_bam_s32k14x/MLIB/bam_f16/MLIB_Convert_F16F32/copyright ==

== system ammclib_bam_s32k14x/MLIB/bam_f16/MLIB_Convert_F16F32/copyright2 ==

== system ammclib_bam_s32k14x/MLIB/bam_f16/MLIB_Convert_F16F32/logo ==

== system ammclib_bam_s32k14x/MLIB/bam_f16/MLIB_Convert_F16FLT/copyright ==

== system ammclib_bam_s32k14x/MLIB/bam_f16/MLIB_Convert_F16FLT/copyright2 ==

== system ammclib_bam_s32k14x/MLIB/bam_f16/MLIB_Convert_F16FLT/logo ==

== system ammclib_bam_s32k14x/MLIB/bam_f16/MLIB_DivSat_F16/copyright ==

== system ammclib_bam_s32k14x/MLIB/bam_f16/MLIB_DivSat_F16/copyright2 ==

== system ammclib_bam_s32k14x/MLIB/bam_f16/MLIB_DivSat_F16/logo ==

== system ammclib_bam_s32k14x/MLIB/bam_f16/MLIB_Div_F16/copyright ==

== system ammclib_bam_s32k14x/MLIB/bam_f16/MLIB_Div_F16/copyright2 ==

== system ammclib_bam_s32k14x/MLIB/bam_f16/MLIB_Div_F16/logo ==

== system ammclib_bam_s32k14x/MLIB/bam_f16/MLIB_MacSat_F16/copyright ==

== system ammclib_bam_s32k14x/MLIB/bam_f16/MLIB_MacSat_F16/copyright2 ==

== system ammclib_bam_s32k14x/MLIB/bam_f16/MLIB_MacSat_F16/logo ==

== system ammclib_bam_s32k14x/MLIB/bam_f16/MLIB_Mac_F16/copyright ==

== system ammclib_bam_s32k14x/MLIB/bam_f16/MLIB_Mac_F16/copyright2 ==

== system ammclib_bam_s32k14x/MLIB/bam_f16/MLIB_Mac_F16/logo ==

== system ammclib_bam_s32k14x/MLIB/bam_f16/MLIB_Mnac_F16/copyright ==

== system ammclib_bam_s32k14x/MLIB/bam_f16/MLIB_Mnac_F16/copyright2 ==

== system ammclib_bam_s32k14x/MLIB/bam_f16/MLIB_Mnac_F16/logo ==

== system ammclib_bam_s32k14x/MLIB/bam_f16/MLIB_Msu_F16/copyright ==

== system ammclib_bam_s32k14x/MLIB/bam_f16/MLIB_Msu_F16/copyright2 ==

== system ammclib_bam_s32k14x/MLIB/bam_f16/MLIB_Msu_F16/logo ==

== system ammclib_bam_s32k14x/MLIB/bam_f16/MLIB_MulSat_F16/copyright ==

== system ammclib_bam_s32k14x/MLIB/bam_f16/MLIB_MulSat_F16/copyright2 ==

== system ammclib_bam_s32k14x/MLIB/bam_f16/MLIB_MulSat_F16/logo ==

== system ammclib_bam_s32k14x/MLIB/bam_f16/MLIB_Mul_F16/copyright ==

== system ammclib_bam_s32k14x/MLIB/bam_f16/MLIB_Mul_F16/copyright2 ==

== system ammclib_bam_s32k14x/MLIB/bam_f16/MLIB_Mul_F16/logo ==

== system ammclib_bam_s32k14x/MLIB/bam_f16/MLIB_NegSat_F16/copyright ==

== system ammclib_bam_s32k14x/MLIB/bam_f16/MLIB_NegSat_F16/copyright2 ==

== system ammclib_bam_s32k14x/MLIB/bam_f16/MLIB_NegSat_F16/logo ==

== system ammclib_bam_s32k14x/MLIB/bam_f16/MLIB_Neg_F16/copyright ==

== system ammclib_bam_s32k14x/MLIB/bam_f16/MLIB_Neg_F16/copyright2 ==

== system ammclib_bam_s32k14x/MLIB/bam_f16/MLIB_Neg_F16/logo ==

== system ammclib_bam_s32k14x/MLIB/bam_f16/MLIB_Norm_F16/copyright ==

== system ammclib_bam_s32k14x/MLIB/bam_f16/MLIB_Norm_F16/copyright2 ==

== system ammclib_bam_s32k14x/MLIB/bam_f16/MLIB_Norm_F16/logo ==

== system ammclib_bam_s32k14x/MLIB/bam_f16/MLIB_RndSat_F16F32/copyright ==

== system ammclib_bam_s32k14x/MLIB/bam_f16/MLIB_RndSat_F16F32/copyright2 ==

== system ammclib_bam_s32k14x/MLIB/bam_f16/MLIB_RndSat_F16F32/logo ==

== system ammclib_bam_s32k14x/MLIB/bam_f16/MLIB_Round_F16/copyright ==

== system ammclib_bam_s32k14x/MLIB/bam_f16/MLIB_Round_F16/copyright2 ==

== system ammclib_bam_s32k14x/MLIB/bam_f16/MLIB_Round_F16/logo ==

== system ammclib_bam_s32k14x/MLIB/bam_f16/MLIB_ShBiSat_F16/copyright ==

== system ammclib_bam_s32k14x/MLIB/bam_f16/MLIB_ShBiSat_F16/copyright2 ==

== system ammclib_bam_s32k14x/MLIB/bam_f16/MLIB_ShBiSat_F16/logo ==

== system ammclib_bam_s32k14x/MLIB/bam_f16/MLIB_ShBi_F16/copyright ==

== system ammclib_bam_s32k14x/MLIB/bam_f16/MLIB_ShBi_F16/copyright2 ==

== system ammclib_bam_s32k14x/MLIB/bam_f16/MLIB_ShBi_F16/logo ==

== system ammclib_bam_s32k14x/MLIB/bam_f16/MLIB_ShLSat_F16/copyright ==

== system ammclib_bam_s32k14x/MLIB/bam_f16/MLIB_ShLSat_F16/copyright2 ==

== system ammclib_bam_s32k14x/MLIB/bam_f16/MLIB_ShLSat_F16/logo ==

== system ammclib_bam_s32k14x/MLIB/bam_f16/MLIB_ShL_F16/copyright ==

== system ammclib_bam_s32k14x/MLIB/bam_f16/MLIB_ShL_F16/copyright2 ==

== system ammclib_bam_s32k14x/MLIB/bam_f16/MLIB_ShL_F16/logo ==

== system ammclib_bam_s32k14x/MLIB/bam_f16/MLIB_ShR_F16/copyright ==

== system ammclib_bam_s32k14x/MLIB/bam_f16/MLIB_ShR_F16/copyright2 ==

== system ammclib_bam_s32k14x/MLIB/bam_f16/MLIB_ShR_F16/logo ==

== system ammclib_bam_s32k14x/MLIB/bam_f16/MLIB_SubSat_F16/copyright ==

== system ammclib_bam_s32k14x/MLIB/bam_f16/MLIB_SubSat_F16/copyright2 ==

== system ammclib_bam_s32k14x/MLIB/bam_f16/MLIB_SubSat_F16/logo ==

== system ammclib_bam_s32k14x/MLIB/bam_f16/MLIB_Sub_F16/copyright ==

== system ammclib_bam_s32k14x/MLIB/bam_f16/MLIB_Sub_F16/copyright2 ==

== system ammclib_bam_s32k14x/MLIB/bam_f16/MLIB_Sub_F16/logo ==

== system ammclib_bam_s32k14x/MLIB/bam_f16/MLIB_VMac_F16/copyright ==

== system ammclib_bam_s32k14x/MLIB/bam_f16/MLIB_VMac_F16/copyright2 ==

== system ammclib_bam_s32k14x/MLIB/bam_f16/MLIB_VMac_F16/logo ==

== system ammclib_bam_s32k14x/MLIB/bam_f32/MLIB_AbsSat_F32/copyright ==

== system ammclib_bam_s32k14x/MLIB/bam_f32/MLIB_AbsSat_F32/copyright2 ==

== system ammclib_bam_s32k14x/MLIB/bam_f32/MLIB_AbsSat_F32/logo ==

== system ammclib_bam_s32k14x/MLIB/bam_f32/MLIB_Abs_F32/copyright ==

== system ammclib_bam_s32k14x/MLIB/bam_f32/MLIB_Abs_F32/copyright2 ==

== system ammclib_bam_s32k14x/MLIB/bam_f32/MLIB_Abs_F32/logo ==

== system ammclib_bam_s32k14x/MLIB/bam_f32/MLIB_AddSat_F32/copyright ==

== system ammclib_bam_s32k14x/MLIB/bam_f32/MLIB_AddSat_F32/copyright2 ==

== system ammclib_bam_s32k14x/MLIB/bam_f32/MLIB_AddSat_F32/logo ==

== system ammclib_bam_s32k14x/MLIB/bam_f32/MLIB_Add_F32/copyright ==

== system ammclib_bam_s32k14x/MLIB/bam_f32/MLIB_Add_F32/copyright2 ==

== system ammclib_bam_s32k14x/MLIB/bam_f32/MLIB_Add_F32/logo ==

== system ammclib_bam_s32k14x/MLIB/bam_f32/MLIB_ConvertPU_F32F16/copyright ==

== system ammclib_bam_s32k14x/MLIB/bam_f32/MLIB_ConvertPU_F32F16/copyright2 ==

== system ammclib_bam_s32k14x/MLIB/bam_f32/MLIB_ConvertPU_F32F16/logo ==

== system ammclib_bam_s32k14x/MLIB/bam_f32/MLIB_ConvertPU_F32FLT/copyright ==

== system ammclib_bam_s32k14x/MLIB/bam_f32/MLIB_ConvertPU_F32FLT/copyright2 ==

== system ammclib_bam_s32k14x/MLIB/bam_f32/MLIB_ConvertPU_F32FLT/logo ==

== system ammclib_bam_s32k14x/MLIB/bam_f32/MLIB_Convert_F32F16/copyright ==

== system ammclib_bam_s32k14x/MLIB/bam_f32/MLIB_Convert_F32F16/copyright2 ==

== system ammclib_bam_s32k14x/MLIB/bam_f32/MLIB_Convert_F32F16/logo ==

== system ammclib_bam_s32k14x/MLIB/bam_f32/MLIB_Convert_F32FLT/copyright ==

== system ammclib_bam_s32k14x/MLIB/bam_f32/MLIB_Convert_F32FLT/copyright2 ==

== system ammclib_bam_s32k14x/MLIB/bam_f32/MLIB_Convert_F32FLT/logo ==

== system ammclib_bam_s32k14x/MLIB/bam_f32/MLIB_DivSat_F32/copyright ==

== system ammclib_bam_s32k14x/MLIB/bam_f32/MLIB_DivSat_F32/copyright2 ==

== system ammclib_bam_s32k14x/MLIB/bam_f32/MLIB_DivSat_F32/logo ==

== system ammclib_bam_s32k14x/MLIB/bam_f32/MLIB_Div_F32/copyright ==

== system ammclib_bam_s32k14x/MLIB/bam_f32/MLIB_Div_F32/copyright2 ==

== system ammclib_bam_s32k14x/MLIB/bam_f32/MLIB_Div_F32/logo ==

== system ammclib_bam_s32k14x/MLIB/bam_f32/MLIB_MacSat_F32/copyright ==

== system ammclib_bam_s32k14x/MLIB/bam_f32/MLIB_MacSat_F32/copyright2 ==

== system ammclib_bam_s32k14x/MLIB/bam_f32/MLIB_MacSat_F32/logo ==

== system ammclib_bam_s32k14x/MLIB/bam_f32/MLIB_Mac_F32/copyright ==

== system ammclib_bam_s32k14x/MLIB/bam_f32/MLIB_Mac_F32/copyright2 ==

== system ammclib_bam_s32k14x/MLIB/bam_f32/MLIB_Mac_F32/logo ==

== system ammclib_bam_s32k14x/MLIB/bam_f32/MLIB_Mnac_F32/copyright ==

== system ammclib_bam_s32k14x/MLIB/bam_f32/MLIB_Mnac_F32/copyright2 ==

== system ammclib_bam_s32k14x/MLIB/bam_f32/MLIB_Mnac_F32/logo ==

== system ammclib_bam_s32k14x/MLIB/bam_f32/MLIB_Msu_F32/copyright ==

== system ammclib_bam_s32k14x/MLIB/bam_f32/MLIB_Msu_F32/copyright2 ==

== system ammclib_bam_s32k14x/MLIB/bam_f32/MLIB_Msu_F32/logo ==

== system ammclib_bam_s32k14x/MLIB/bam_f32/MLIB_MulSat_F32/copyright ==

== system ammclib_bam_s32k14x/MLIB/bam_f32/MLIB_MulSat_F32/copyright2 ==

== system ammclib_bam_s32k14x/MLIB/bam_f32/MLIB_MulSat_F32/logo ==

== system ammclib_bam_s32k14x/MLIB/bam_f32/MLIB_Mul_F32/copyright ==

== system ammclib_bam_s32k14x/MLIB/bam_f32/MLIB_Mul_F32/copyright2 ==

== system ammclib_bam_s32k14x/MLIB/bam_f32/MLIB_Mul_F32/logo ==

== system ammclib_bam_s32k14x/MLIB/bam_f32/MLIB_NegSat_F32/copyright ==

== system ammclib_bam_s32k14x/MLIB/bam_f32/MLIB_NegSat_F32/copyright2 ==

== system ammclib_bam_s32k14x/MLIB/bam_f32/MLIB_NegSat_F32/logo ==

== system ammclib_bam_s32k14x/MLIB/bam_f32/MLIB_Neg_F32/copyright ==

== system ammclib_bam_s32k14x/MLIB/bam_f32/MLIB_Neg_F32/copyright2 ==

== system ammclib_bam_s32k14x/MLIB/bam_f32/MLIB_Neg_F32/logo ==

== system ammclib_bam_s32k14x/MLIB/bam_f32/MLIB_Norm_F32/copyright ==

== system ammclib_bam_s32k14x/MLIB/bam_f32/MLIB_Norm_F32/copyright2 ==

== system ammclib_bam_s32k14x/MLIB/bam_f32/MLIB_Norm_F32/logo ==

== system ammclib_bam_s32k14x/MLIB/bam_f32/MLIB_Round_F32/copyright ==

== system ammclib_bam_s32k14x/MLIB/bam_f32/MLIB_Round_F32/copyright2 ==

== system ammclib_bam_s32k14x/MLIB/bam_f32/MLIB_Round_F32/logo ==

== system ammclib_bam_s32k14x/MLIB/bam_f32/MLIB_ShBiSat_F32/copyright ==

== system ammclib_bam_s32k14x/MLIB/bam_f32/MLIB_ShBiSat_F32/copyright2 ==

== system ammclib_bam_s32k14x/MLIB/bam_f32/MLIB_ShBiSat_F32/logo ==

== system ammclib_bam_s32k14x/MLIB/bam_f32/MLIB_ShBi_F32/copyright ==

== system ammclib_bam_s32k14x/MLIB/bam_f32/MLIB_ShBi_F32/copyright2 ==

== system ammclib_bam_s32k14x/MLIB/bam_f32/MLIB_ShBi_F32/logo ==

== system ammclib_bam_s32k14x/MLIB/bam_f32/MLIB_ShLSat_F32/copyright ==

== system ammclib_bam_s32k14x/MLIB/bam_f32/MLIB_ShLSat_F32/copyright2 ==

== system ammclib_bam_s32k14x/MLIB/bam_f32/MLIB_ShLSat_F32/logo ==

== system ammclib_bam_s32k14x/MLIB/bam_f32/MLIB_ShL_F32/copyright ==

== system ammclib_bam_s32k14x/MLIB/bam_f32/MLIB_ShL_F32/copyright2 ==

== system ammclib_bam_s32k14x/MLIB/bam_f32/MLIB_ShL_F32/logo ==

== system ammclib_bam_s32k14x/MLIB/bam_f32/MLIB_ShR_F32/copyright ==

== system ammclib_bam_s32k14x/MLIB/bam_f32/MLIB_ShR_F32/copyright2 ==

== system ammclib_bam_s32k14x/MLIB/bam_f32/MLIB_ShR_F32/logo ==

== system ammclib_bam_s32k14x/MLIB/bam_f32/MLIB_SubSat_F32/copyright ==

== system ammclib_bam_s32k14x/MLIB/bam_f32/MLIB_SubSat_F32/copyright2 ==

== system ammclib_bam_s32k14x/MLIB/bam_f32/MLIB_SubSat_F32/logo ==

== system ammclib_bam_s32k14x/MLIB/bam_f32/MLIB_Sub_F32/copyright ==

== system ammclib_bam_s32k14x/MLIB/bam_f32/MLIB_Sub_F32/copyright2 ==

== system ammclib_bam_s32k14x/MLIB/bam_f32/MLIB_Sub_F32/logo ==

== system ammclib_bam_s32k14x/MLIB/bam_f32/MLIB_VMac_F32/copyright ==

== system ammclib_bam_s32k14x/MLIB/bam_f32/MLIB_VMac_F32/copyright2 ==

== system ammclib_bam_s32k14x/MLIB/bam_f32/MLIB_VMac_F32/logo ==

== system ammclib_bam_s32k14x/MLIB/bam_f32f16f16/MLIB_MacSat_F32F16F16/copyright ==

== system ammclib_bam_s32k14x/MLIB/bam_f32f16f16/MLIB_MacSat_F32F16F16/copyright2 ==

== system ammclib_bam_s32k14x/MLIB/bam_f32f16f16/MLIB_MacSat_F32F16F16/logo ==

== system ammclib_bam_s32k14x/MLIB/bam_f32f16f16/MLIB_Mac_F32F16F16/copyright ==

== system ammclib_bam_s32k14x/MLIB/bam_f32f16f16/MLIB_Mac_F32F16F16/copyright2 ==

== system ammclib_bam_s32k14x/MLIB/bam_f32f16f16/MLIB_Mac_F32F16F16/logo ==

== system ammclib_bam_s32k14x/MLIB/bam_f32f16f16/MLIB_Mnac_F32F16F16/copyright ==

== system ammclib_bam_s32k14x/MLIB/bam_f32f16f16/MLIB_Mnac_F32F16F16/copyright2 ==

== system ammclib_bam_s32k14x/MLIB/bam_f32f16f16/MLIB_Mnac_F32F16F16/logo ==

== system ammclib_bam_s32k14x/MLIB/bam_f32f16f16/MLIB_Msu_F32F16F16/copyright ==
